simulink model "boost_and_two_level__1_sm_ehs"  (Simulink 8.4)
settings: Solver=ode3  SolverMode=SingleTasking  StartTime=0.0  StopTime=inf  FixedStep=2e-05  RelTol=1e-3
PostLoadFcn:
  | Ts = 20e-6;
InitFcn:
  | Ts = 20e-6;
undefined symbols (not defined in the file or in its folder): another_event_name, my_event_name, SW01
libraries: powerlib_meascontrol x12, opal_lib x7, rteventslib x6, rtlab x4, simulink x3, cpuhilios_lib x3, rtio_opalrt_common x2, artemis x1, simulink_extras x1, cpuconverter_lib x1
settings Model: ARTEMISmethode_block_infos=$$__separator__$$boost_and_two_level__1_sm_ehs/ARTEMIS Guide$$__separator__$$  Creator=PYRobert  LastModifiedBy=jiang  BufferReuse=off
settings DataIOCC: SaveOutput=off  SignalLogging=off  SaveTime=off  SignalLoggingName=sigsOut
settings OptimizationCC: BlockReduction=off  OptimizeBlockIOStorage=off  BufferReuse=off  GlobalBufferReuse=off  ExpressionFolding=off  LocalBlockOutputs=off  InitFltsAndDblsToZero=on
settings DebuggingCC: SaveWithParameterizedLinksMsg=none  SignalResolutionControl=TryResolveAllWithWarning  SolverPrmCheckMsg=none  MultiTaskDSMMsg=warning  MultiTaskCondExecSysMsg=none
settings HardwareCC: TargetEndianess=LittleEndian  TargetHWDeviceType=MATLAB Host  ProdEqTarget=off
settings RTWCC: GenCodeOnly=on  IncludeERTFirstTime=on
settings GRTTargetCC: TargetFcnLib=ansi_tfl_tmw.mat
settings ConfigurationSet: Description=SimMechanics 2G

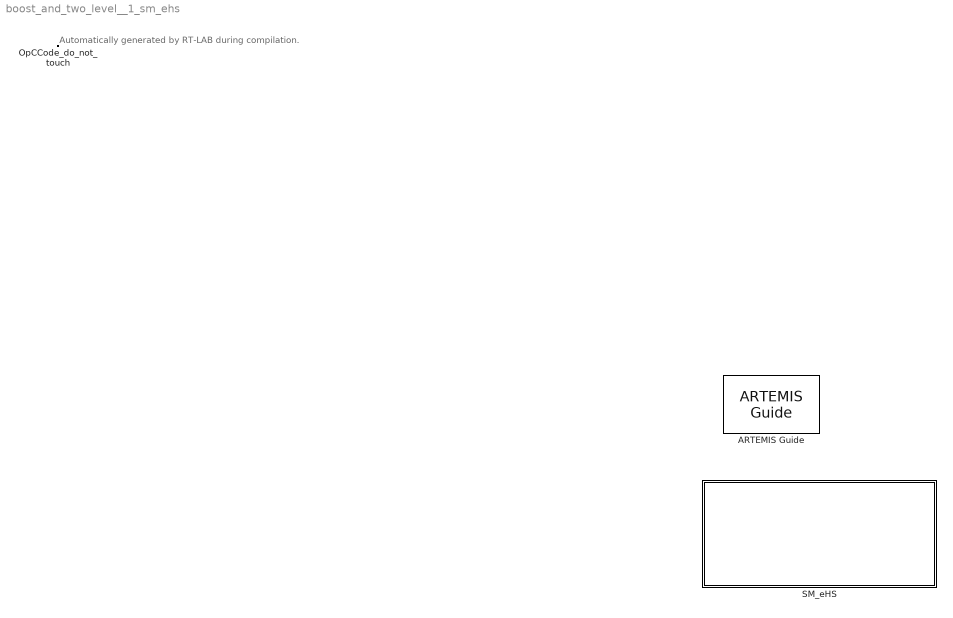
== system boost_and_two_level__1_sm_ehs ==
  note: Automatically generated by RT-LAB during compilation.
  ARTEMIS Guide : artemis/ARTEMIS/ARTEMIS Guide  Tag=FTSSmethode_opal_4hx0r99  Description=5.0_z1  lock=on  Ts=Ts  opt=art5  dyna=off  nb_perm=4  RT_fullcomp=off  ssn=on  ssn_itvc=off  ssn_ivic=off  ssn_ext=off  ssn_solver=Art5 with Backward Euler nodal interface  ssn_impulse=off  ssn_quasimpulse=off  ssn_impulse_loop=5  paraExtinctionThy=off  Thy_Impulse=on  dtc=Off  dtc_opt=normal  ao=on  simtype=off  ct_mac=off  lin_mov=off  lsp=[0.001 2]  spike_skip=Disabled  dtc_extra=1  dtc_sws=normal  dtc_pied=0.5  SPSRulesBlock=SPSRules  tre=on  ctmm=off  LF=off  dpl_type=ARTEMiS DPL  rlc_type=off  custom_type=off  para=on  ssn_ImpulseLoopBlockedStateUpdate=5  ssn_mov_iter_number=5  ssn_switch_iter_number=5
  OpCCode_do_not_touch : opal_lib/Communication/OpCCode  SystemSampleTime=-1
  SM_eHS : Subsystem

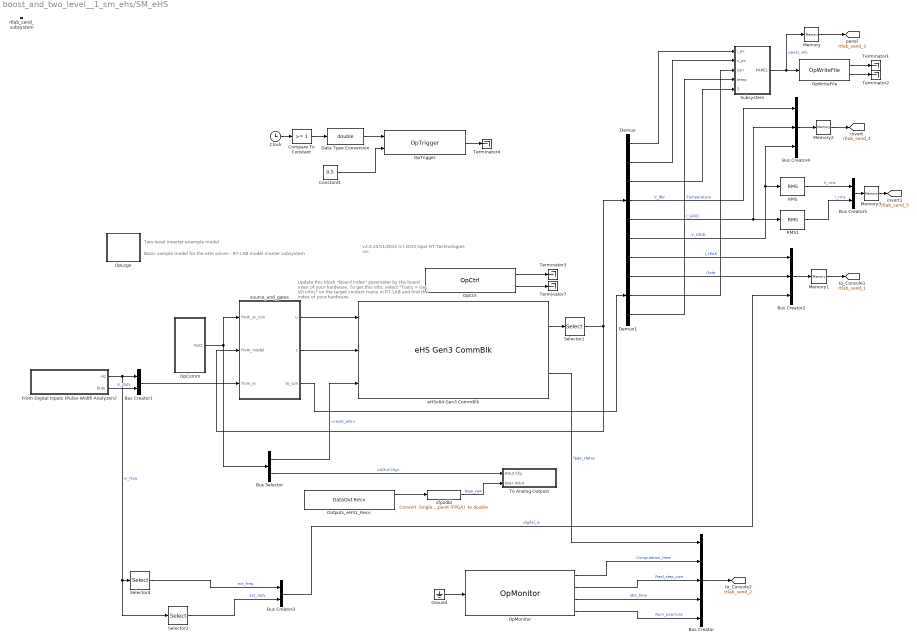
== system boost_and_two_level__1_sm_ehs/SM_eHS ==
  note: v2.0 25/11/2015
      | (c) 2015 Opal-RT Technologies inc.
  note: Two-level inverter example model
  note: Basic sample model for the eHS solver - RT-LAB model master subsystem
  note: Update this block "Board Index" parameter by the
      | board intex of your hardware. To get this info, select
      | "Tools > Get I/O infos" on the target context menu
      | in RT-LAB and find the index of your hardware.
  Bus Creator : BusCreator  Inputs=5
  Bus Creator1 : BusCreator  Inputs=2
  Bus Creator2 : BusCreator  Inputs=3
  Bus Creator3 : BusCreator  Inputs=2
  Bus Creator4 : BusCreator  Inputs=3
  Bus Creator5 : BusCreator  Inputs=2
  Bus Selector : BusSelector  OutputSignals=reset_ehs,AOut Cfg
  Clock : Clock
  Compare To Constant : simulink/Logic and Bit Operations/Compare To Constant  relop=>=  const=1  OutDataTypeStr=boolean
  Constant1 : Constant  Value=0.5
  Data Type Conversion : DataTypeConversion  OutDataTypeStr=double
  Demux : Demux  Outputs=7
  Demux1 : Demux  Outputs=3
  From Digital Inputs (Pulse-Width Analyzers) : Subsystem
  Ground : Ground
  Memory{,1..3} (4 alike) : Memory
  OpComm : Subsystem
      mask init:
      | opmaskdisplay('maskdisplay_block',gcb,'disp(''OpComm'')');
      mask Display:
      | patch([0 0.5 0.7 0],[1 1 0 0],[0.7 0.75 0.9]);
      | patch([1 0.53 0.73 1],[1 1 0 0],[1 0.8 0.7]);
      | plot([0 0 1 1 0],[0 1 1 0 0]);
      | disp('OpComm')
  OpCtrl : rtio_opalrt_common/OpCtrl  CtrlName='OpCtrl'  boardid=0  BitstreamFilename=MMPK7_1-EX-0001-2_3_2_19-300Series_eHSgen3_with_IOs-303-03.bin  numconfig=-1  mode=Master  externalClock=off  decimRtsi=0  calibIO=off  SampleTime=0  loadinport=-1  BoardType=MMPK7  SecondaryPresent=off  sync_type=Audio
  OpLogo : Subsystem
      mask Display:
      | opLogo = imread('efsOpLogo.tif','tif');
      | image(opLogo(:,:,1:3));
  OpMonitor : rtlab/Monitoring/OpMonitor  compute_time=on  real_step=on  idle_time=on  nb_overruns=on  user_time=off  user_name=my_event_name,another_event_name
  OpTrigger : rtlab/DataLogging/OpTrigger  Trig_Type=RISING OR FALLING EDGE  Trig_Offset=0  Acq_Group=26
  OpWriteFile : rtlab/DataLogging/OpWriteFile  Static_File=on  varname=opvar  Filename=myPV_inverter.mat  rtpath='./'  nrtpath='.\'  Acq_Group=26  file_size=1024*1024*1024  write_offline=off  Sim_Mode=off  Nb_Samples=4e5  Buffer_size=1024*1024
      settings: Decimation=100
  Outputs_eHS1_Recv : rtio_opalrt_common/DataOut Recv  CtrlName='OpCtrl'  FcnNos=2  width=7  portType=uint32  sampleTime=0  checkVersion=off  expectedId=0  expectedVersion=0  opComp=>=
      settings: AttributesFormatString=%<CtrlName>
  RMS : powerlib_meascontrol/Measurements/RMS  TrueRMS=on  Freq=50  RMSInit=0  Ts=0
  RMS1 : powerlib_meascontrol/Measurements/RMS  TrueRMS=on  Freq=50  RMSInit=0  Ts=0
  Selector1 : Selector  Indices=[1:7]
  Selector2 : Selector  InputPortWidth=2  Indices=[2]
  Selector4 : Selector  InputPortWidth=2  Indices=[1]
  Subsystem : Subsystem
  Terminator{1..4,7} (5 alike) : Terminator
  To Analog Outputs : Subsystem
  eHSx64 Gen3 CommBlk : cpuconverter_lib/eHS Gen3 CommBlk  GenMat=off  solver_size=x64  circuit_mtx1=my_pv_sys_fpga.mdl  Ts_eHS_1_explicit=on  Ts_eHS_1=2.5e-07  SimeHS1=off  ShowAdv1=on  gs1=0.076389  v_init1=400*ones(1,24)  i_init1=zeros(1,24)  netlist_name=my_pv_sys_fpga.mdl  ts_min=2.05e-07  nb_u=3  input_names=|  nb_sw=4  switches_names=SW01-04_01 | SW01-04_02 | SW01-04_03 | SW01-04_04  nb_y=7  output_names=Y01 IPANEL I | Y02 VPANEL U | Y03 VPH U | Y04 VINV U | Y05 IGRID I | Y06 VGRID U | Y07 IG I  nb_nsd=12  Input_config1_popup=Constant from RT-LAB block (all)  input_config_1="[zeros(32,1)  (0:31)']"  input_nb_auto=on  input_nb=3  UseSWG=off  SWGPortNbs=3  Pulse_ctrl1_popup=Independent setting for each element  GateCtrlSelPanel=off  Pulse_ctrl1=[zeros(72,1) (0:71)']  Polarity1_popup=Active-high (all)  Polarity1=zeros(1,72)  pulse_nb=8  rte_pulse_nb=SW01-08  nb_event=4  static_pulse=none  scn_en=off  xls_file=diode_bridge.xls  scn_cmd=do nothing  xls_page=1  nscn_max=102  nscn_used=1  scn_log_en=on  CtrlName='OpCtrl'  Ts=Ts  PortNbs=[1 2 1 2:1:2+8 1]  blkid1=0
      | U01
      | 14,400 V | U02 IPH
      |  | U03 ID
      settings: AttributesFormatString=%<CtrlName>
  rtlab_send_subsystem : Subsystem  Priority=-100
      mask Display: text(0,0,'');
  sfp2dbl : rtlab/Miscellaneous/Convert  Single floating-point (FPGA)  to double
  source_and_gates : Subsystem
  tag scope: rtlab_send_1=global, rtlab_send_2=global, rtlab_send_3=global, rtlab_send_4=global, rtlab_send_5=global
  wires:
  OpComm/1(Out1) -> Bus Selector/1, source_and_gates/1(from_sc_con)
  OpCtrl/1 -> Terminator3/1
  OpCtrl/2 -> Terminator7/1
  source_and_gates/1(u) -> eHSx64 Gen3 CommBlk/1
  source_and_gates/2(c) -> eHSx64 Gen3 CommBlk/2
  eHSx64 Gen3 CommBlk/1 -> Selector1/1
  Outputs_eHS1_Recv/1 -> sfp2dbl/1
  Bus Selector/1 -> eHSx64 Gen3 CommBlk/3  "<reset_ehs>"
  Selector1/1 -> Demux/1, source_and_gates/2(from_model)
  OpWriteFile/1 -> Terminator1/1
  OpWriteFile/2 -> Terminator2/1
  Clock/1 -> Compare To Constant/1
  Constant1/1 -> OpTrigger/2
  OpTrigger/1 -> Terminator4/1
  Compare To Constant/1 -> Data Type Conversion/1
  Data Type Conversion/1 -> OpTrigger/1
  Ground/1 -> OpMonitor/1
  Bus Creator/1 -> [rtlab_send_2]
  sfp2dbl/1 -> To Analog Outputs/2(User AOut)  "fpga_raw"
  OpMonitor/4 -> Bus Creator/5  "Num_overruns"
  OpMonitor/3 -> Bus Creator/4  "Idle_time"
  OpMonitor/2 -> Bus Creator/3  "Real_step_size"
  OpMonitor/1 -> Bus Creator/2  "Computation_time"
  Subsystem/1(PANEL) -> Memory/1, OpWriteFile/1  "panel_info"
  Bus Selector/2 -> To Analog Outputs/1(AOut Cfg)  "<AOut Cfg>"
  Demux/1 -> Subsystem/1(i_pv)
  Demux/2 -> Subsystem/2(v_pv)
  Demux/4 -> Bus Creator4/1  "V_INV"
  Demux/3 -> Subsystem/5(i_diode)
  Demux/5 -> RMS1/1, Bus Creator4/2  "I_GRID"
  Demux/6 -> RMS/1, Bus Creator4/3  "V_GRID"
  Demux/7 -> Bus Creator2/1  "I_LEAK"
  source_and_gates/3(to_con) -> Demux1/1
  Demux1/3 -> Subsystem/4(temp)  "Temperature"
  Demux1/1 -> Bus Creator2/2  "Gate"
  Demux1/2 -> Subsystem/3(sun)
  Bus Creator2/1 -> Memory1/1
  From Digital Inputs (Pulse-Width Analyzers)/1(Hz) -> Selector2/1, Selector4/1, Bus Creator1/1  "in_freq"
  From Digital Inputs (Pulse-Width Analyzers)/2(Duty) -> Bus Creator1/2  "in_duty"
  Bus Creator1/1 -> source_and_gates/3(from_io)
  Selector4/1 -> Bus Creator3/1  "ext_freq"
  Bus Creator3/1 -> Bus Creator2/3  "digital_in"
  eHSx64 Gen3 CommBlk/2 -> Bus Creator/1  "fpga_status"
  Memory/1 -> [rtlab_send_3]
  Memory1/1 -> [rtlab_send_1]
  Memory2/1 -> [rtlab_send_4]
  Bus Creator4/1 -> Memory2/1
  RMS/1 -> Bus Creator5/1  "V_rms"
  RMS1/1 -> Bus Creator5/2  "I_rms"
  Bus Creator5/1 -> Memory3/1
  Memory3/1 -> [rtlab_send_5]
  Selector2/1 -> Bus Creator3/2  "ext_duty"

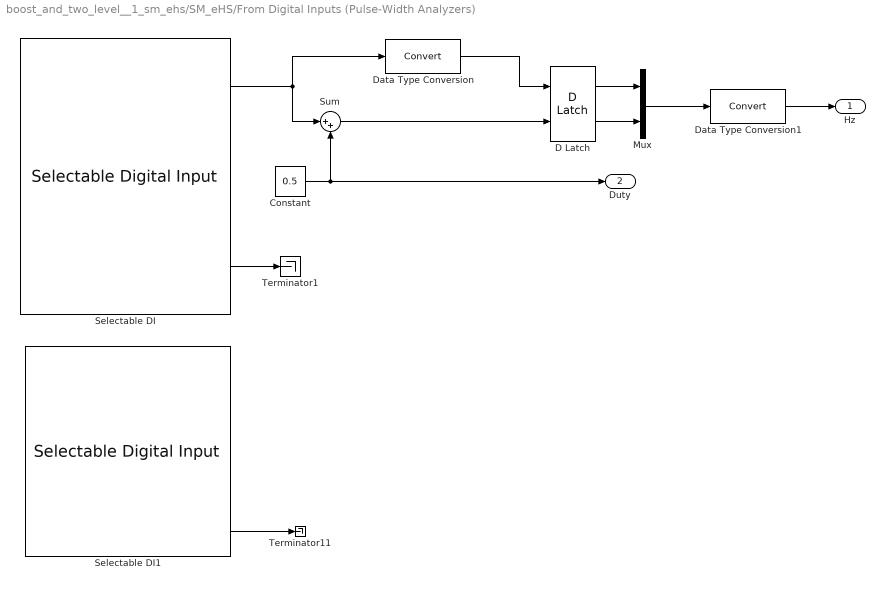
== system boost_and_two_level__1_sm_ehs/SM_eHS/From Digital Inputs (Pulse-Width Analyzers) ==
  Constant : Constant  Value=0.5
  D Latch : simulink_extras/Flip Flops/D Latch
  Data Type Conversion : DataTypeConversion
  Data Type Conversion1 : DataTypeConversion
  Mux : Mux  Inputs=2
  Selectable DI : cpuhilios_lib/Selectable Digital Input  CtrlName='OpCtrl'  DataInPortNumber=5  LoadInPortNumber=13  IOTypeSel=Event Detector  FcnNos=Slot 1 Module A Subsection 1  maxcount=8  count=1  width=1  timeUnit=Time ratio  sampleTime=0
      settings: AttributesFormatString=%<CtrlName>
  Selectable DI1 : cpuhilios_lib/Selectable Digital Input  CtrlName='OpCtrl'  DataInPortNumber=6  LoadInPortNumber=14  IOTypeSel=Event Detector  FcnNos=Slot 1 Module A Subsection 2  maxcount=8  count=8  width=0  timeUnit=Time ratio  sampleTime=0
      settings: AttributesFormatString=%<CtrlName>
  Sum : Sum  Inputs=|++
  Terminator1 : Terminator
  Terminator11 : Terminator
  Hz : Outport
  Duty : Outport  Port=2
  wires:
  Selectable DI1/17 -> Terminator11/1
  Selectable DI/3 -> Terminator1/1
  D Latch/1 -> Mux/1
  D Latch/2 -> Mux/2
  Mux/1 -> Data Type Conversion1/1
  Selectable DI/1 -> Sum/1, Data Type Conversion/1
  Constant/1 -> Duty/1, Sum/2
  Data Type Conversion/1 -> D Latch/1
  Sum/1 -> D Latch/2
  Data Type Conversion1/1 -> Hz/1

== system boost_and_two_level__1_sm_ehs/SM_eHS/OpComm ==
  Demux : Demux  Outputs=[165]
  Receive : opal_lib/Communication/OpRecPar FromNT  Data_width=165  InitialConditions=[1000;25;1;0;49;48;52;53;53;9;1;3;12;13;0;2;48;49;50;51;48;49;50;51;52;53;54;54;56;57;58;59;60;61;62;63;0.0066;0.33;0.066;0.004125;0.0048529;1;0.005;0.005;0.1;0.1;0.1;0.1;0.005;0.1;0.1;0.1;1;1;1;1;1;1;1;1;1;1;1;1;1;1;1;1;0;0;1.65;1.65;1.65;0;0;0;0;0;0;0;0;0;0;0;0;0;0;0;0;0;0;0;0;0;0;0;0;0;0;0;3.3;3.3;3.3;3.3;3.3;5;5;5;5;5;5;5;16;16;16;16;16;16;16;16;16;16;16;16;16;16;16;16;16;16;16;16;0;0;0;0;0;-5;-5;-5;-5;-5;-5;-5;-16;-16;-16;-16;-16;-16;-16;-16;-16;-16;-16;-16;-16;-16;-16;-16;-16;-16;-16;-16;2]
  busStruct : Subsystem
  Out1 : Outport
  wires:
  Demux/1 -> busStruct/1(In1)
  busStruct/1(Out1) -> Out1/1
  Receive/1 -> Demux/1

== system boost_and_two_level__1_sm_ehs/SM_eHS/OpLogo ==

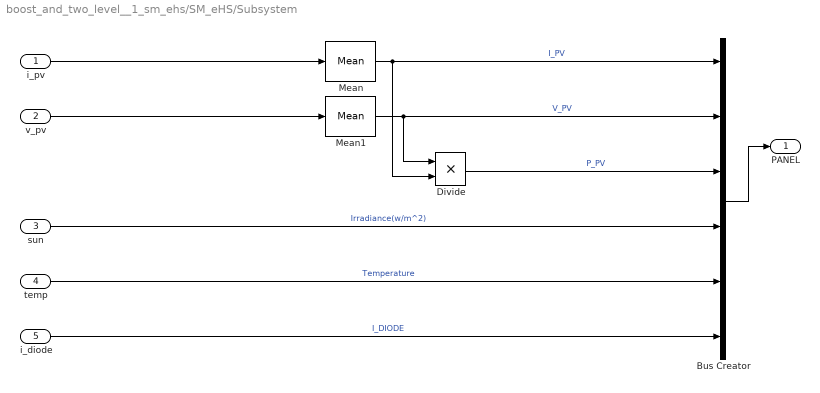
== system boost_and_two_level__1_sm_ehs/SM_eHS/Subsystem ==
  i_pv : Inport
  v_pv : Inport  Port=2
  sun : Inport  Port=3
  temp : Inport  Port=4
  i_diode : Inport  Port=5
  Bus Creator : BusCreator  Inputs=6
  Divide : Product  Inputs=**
  Mean : powerlib_meascontrol/Measurements/Mean  Freq=50  Vinit=0  Ts=0
  Mean1 : powerlib_meascontrol/Measurements/Mean  Freq=50  Vinit=0  Ts=0
  PANEL : Outport
  wires:
  Divide/1 -> Bus Creator/3  "P_PV"
  Mean/1 -> Divide/2, Bus Creator/1  "I_PV"
  Mean1/1 -> Divide/1, Bus Creator/2  "V_PV"
  sun/1 -> Bus Creator/4  "Irradiance(w/m^2)"
  i_pv/1 -> Mean/1
  v_pv/1 -> Mean1/1
  Bus Creator/1 -> PANEL/1
  temp/1 -> Bus Creator/5  "Temperature"
  i_diode/1 -> Bus Creator/6  "I_DIODE"

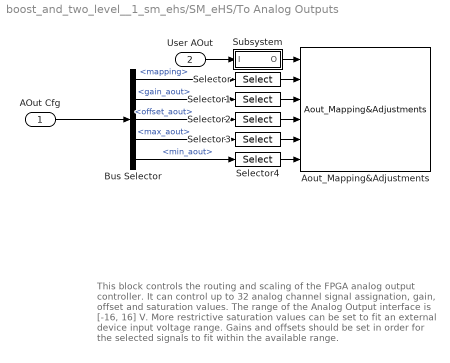
== system boost_and_two_level__1_sm_ehs/SM_eHS/To Analog Outputs ==
  note: This block controls the routing and scaling of the FPGA analog
      | output controller.
      |
      |  It can control up to 32 analog channel signal assignation, gain,
      | offset and saturation values.
      |
      | The range of the Analog Output interface is [-16, 16] V.  More
      | restrictive saturation values can be set to fit an external device
      | input voltage range. Gains and offsets should be set in order for
      | the selected signals to fit within the available range.
  AOut Cfg : Inport
  User AOut : Inport  Port=2
  Aout_Mapping&Adjustments : cpuhilios_lib/Aout_Mapping&Adjustments  ChNum=16 (1 Aout mezz)  UserAoutNum=16  block_index=0  DataInId=15  LoadInId=4  CtrlerName='OpCtrl'
      settings: AttributesFormatString=%<CtrlerName>
  Bus Selector : BusSelector  OutputSignals=mapping,gain_aout,offset_aout,max_aout,min_aout
  Selector{,1..4} (5 alike) : Selector  InputPortWidth=32  Indices=[1:1:16]
  Subsystem : Subsystem
  wires:
  User AOut/1 -> Subsystem/1(I)
  Bus Selector/2 -> Selector1/1  "<gain_aout>"
  Bus Selector/5 -> Selector4/1  "<min_aout>"
  Bus Selector/4 -> Selector3/1  "<max_aout>"
  Bus Selector/1 -> Selector/1  "<mapping>"
  Bus Selector/3 -> Selector2/1  "<offset_aout>"
  AOut Cfg/1 -> Bus Selector/1
  Subsystem/1(O) -> Aout_Mapping&Adjustments/1
  Selector/1 -> Aout_Mapping&Adjustments/2
  Selector1/1 -> Aout_Mapping&Adjustments/3
  Selector2/1 -> Aout_Mapping&Adjustments/4
  Selector3/1 -> Aout_Mapping&Adjustments/5
  Selector4/1 -> Aout_Mapping&Adjustments/6

== system boost_and_two_level__1_sm_ehs/SM_eHS/rtlab_send_subsystem ==
  Subsystem1 : Subsystem
  Subsystem2 : Subsystem
  Subsystem3 : Subsystem
  Subsystem4 : Subsystem
  Subsystem5 : Subsystem
  wires:
  [rtlab_send_1] -> Subsystem1/1(In1)
  [rtlab_send_2] -> Subsystem2/1(In1)
  [rtlab_send_4] -> Subsystem3/1(In1)
  [rtlab_send_3] -> Subsystem4/1(In1)
  [rtlab_send_5] -> Subsystem5/1(In1)

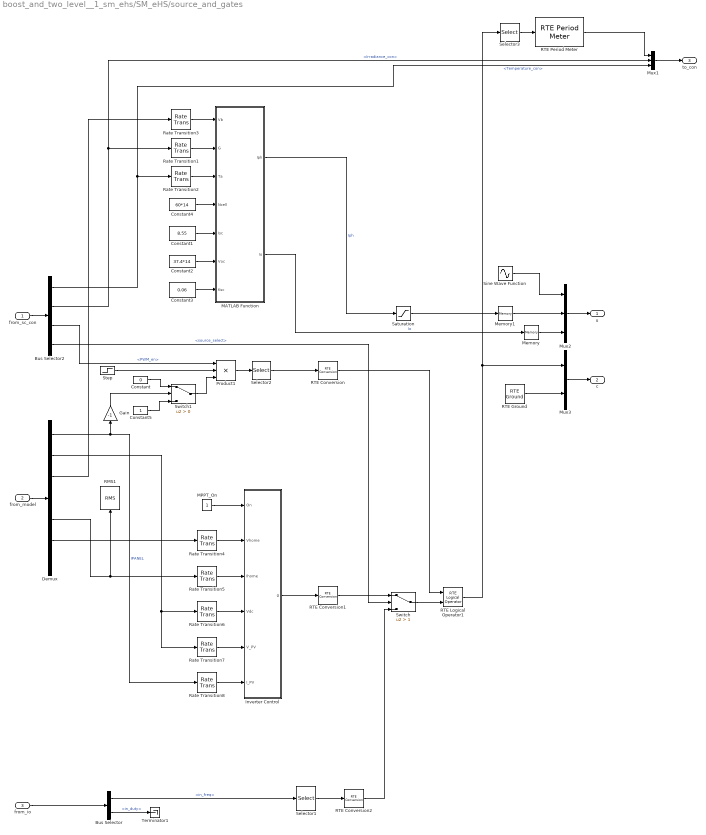
== system boost_and_two_level__1_sm_ehs/SM_eHS/source_and_gates ==
  from_sc_con : Inport
  from_model : Inport  Port=2
  from_io : Inport  Port=3
  Bus Selector : BusSelector  OutputSignals=in_freq,in_duty
  Bus Selector2 : BusSelector  OutputSignals=Temperature_con,Irradiance_con,PWM_en,source_select
  Constant : Constant  Value=0
  Constant1 : Constant  Value=8.55
  Constant2 : Constant  Value=37.4*14
  Constant3 : Constant  Value=0.06
  Constant4 : Constant  Value=60*14
  Constant5 : Constant
  Demux : Demux  Outputs=7
  Gain : Gain  Gain=-1
  Inverter Control : Subsystem  mask(Inverter Control){Pnom=3500, Fnom=50, Vnom_prim=240, Vnom_dc=400, Increment_MPPT=0.003, Limits_MPPT=[ 450 375 ], Vdc_ref_Init=425, Kp_VDCreg=12, Ki_VDCreg=200, Kp_Ireg=0.15, Ki_Ireg=6.6, RLff=[ 0.002 0.20 ], Fc=8000, PWMmode12=Bipolar, Ts_Control=Ts, Ts_PWMgenerator=Ts}
      mask prompts: Pnom "Power (VA)"; Fnom "Frequency (Hz)"; Vnom_prim "Primary voltage (Vrms LL)"; Vnom_dc "DC voltage (V)"; Increment_MPPT "Output increment (V)"; Limits_MPPT "Output limits [ Upper  Lower ]"; Vdc_ref_Init "Output initial value (V)"; Kp_VDCreg "Proportional gain"; Ki_VDCreg "Integral gain"; Kp_Ireg "Proportional gain"; Ki_Ireg "Integral gain"; RLff "Feedforward Values [Rff Lff] (pu)"; Fc "Carrier frequency (Hz)"; PWMmode12 "PWM method"; Ts_Control "Control systems"; Ts_PWMgenerator "PWM generator"
      mask help:
      | The main components of the Inverter Control are:
      | 1. PLL & Measurements
      | 2. Maximum Power Point Tracker System (MPPT) using a Perturb & Observe algorithm
      | 3. DC Voltage Regulator
      | 4. Current Regulator
      | 5. PWM Modulator
      mask TypeOptions PWMmode12: Unipolar | Bipolar
      mask Display:
      | blockName=gcb;
      | if PWMmode12==1
      |     set_param([blockName,'/','PWM_Generator'],'ModulatorType','Single-phase full-bridge (4 pulses)')
      | else
      |     set_param([blockName,'/','PWM_Generator'],'ModulatorType','Single-phase full-bridge - Bipolar modulation (4 pulses)')
      | end
  MATLAB Function : MATLAB Function  TreatAsAtomicUnit=on
  MPPT_On : Constant
  Memory : Memory  InheritSampleTime=on  LinearizeAsDelay=on
  Memory1 : Memory  InheritSampleTime=on  LinearizeAsDelay=on
  Mux1 : Mux  Inputs=3
  Mux2 : Mux  Inputs=3
  Mux3 : Mux  Inputs=2
  Product1 : Product  Inputs=3  RndMeth=Zero
  RMS1 : powerlib_meascontrol/Measurements/RMS  TrueRMS=on  Freq=50  RMSInit=0  Ts=0
  RTE Conversion : rteventslib/Signal Attributes/RTE Conversion  inputdatatype=Double  outputdatatype=RTE Boolean  compensation=Enabled  nbMaxEvents=100  sampleTime=Ts
  RTE Conversion1 : rteventslib/Signal Attributes/RTE Conversion  inputdatatype=Double  outputdatatype=RTE Boolean  compensation=Enabled  nbMaxEvents=4  sampleTime=Ts
  RTE Conversion2 : rteventslib/Signal Attributes/RTE Conversion  inputdatatype=Double  outputdatatype=RTE Boolean  compensation=Enabled  nbMaxEvents=4  sampleTime=Ts
  RTE Ground : rteventslib/Sources/RTE Ground  SampleTime=Ts
  RTE Logical Operator1 : rteventslib/Math Operations/RTE Logical Operator  LogicalOperator=AND  NbrInput=2  NbrMaxEvents=255
  RTE Period Meter : rteventslib/Signal Attributes/RTE Period Meter  Period=off  Frequency=off  EdgeType=Rising edges  TOn=off  TOff=off  DutyCycle=on  DuringType=Signal period  MinimumFrequency=0
  Rate Transition1 : RateTransition  X0=1000
  Rate Transition2 : RateTransition  X0=25
  Rate Transition3 : RateTransition  X0=400
  Rate Transition4 : RateTransition
  Rate Transition5 : RateTransition
  Rate Transition6 : RateTransition  X0=400
  Rate Transition7 : RateTransition  X0=400
  Rate Transition8 : RateTransition
  Saturation : Saturate  UpperLimit=10  LowerLimit=0
  Selector1 : Selector  InputPortWidth=2  Indices=[1 2 2 1]
  Selector2 : Selector  InputPortWidth=1  Indices=[ones(1,4)*1]
  Selector3 : Selector  Indices=[1]
  Sine Wave Function : Sin  Amplitude=14400*sqrt(2)  Frequency=50*2*pi  SampleTime=0
  Step : Step  Time=0.05  SampleTime=Ts
  Switch : Switch  Criteria=u2 > Threshold  Threshold=1
  Switch1 : Switch  Criteria=u2 > Threshold
  Terminator1 : Terminator
  u : Outport
  c : Outport  Port=2
  to_con : Outport  Port=3
  wires:
  Bus Selector2/3 -> Product1/1  "<PWM_en>"
  Step/1 -> Product1/2
  Product1/1 -> Selector2/1
  Mux2/1 -> u/1
  from_sc_con/1 -> Bus Selector2/1
  MPPT_On/1 -> Inverter Control/1(On)
  Constant4/1 -> MATLAB Function/4(Ncell)
  Constant1/1 -> MATLAB Function/5(Isc)
  Constant2/1 -> MATLAB Function/6(Voc)
  Constant3/1 -> MATLAB Function/7(Ksc)
  from_model/1 -> Demux/1
  Demux/1 -> Gain/1, Rate Transition8/1  "IPANEL"
  Demux/2 -> Rate Transition7/1, Rate Transition6/1
  Demux/6 -> Rate Transition4/1
  Demux/5 -> RMS1/1, Rate Transition5/1
  Mux1/1 -> to_con/1
  RTE Ground/1 -> Mux3/2
  Mux3/1 -> c/1
  Sine Wave Function/1 -> Mux2/1
  MATLAB Function/2(Io) -> Memory/1  "Io"
  Saturation/1 -> Memory1/1
  MATLAB Function/1(Iph) -> Saturation/1  "Iph"
  Memory1/1 -> Mux2/2
  Memory/1 -> Mux2/3
  Rate Transition3/1 -> MATLAB Function/1(Vb)
  Rate Transition1/1 -> MATLAB Function/2(G)
  Rate Transition2/1 -> MATLAB Function/3(Ta)
  Bus Selector2/2 -> Mux1/2, Rate Transition1/1  "<Irradiance_con>"
  Bus Selector2/1 -> Rate Transition2/1, Mux1/3  "<Temperature_con>"
  Demux/3 -> Rate Transition3/1
  Rate Transition4/1 -> Inverter Control/2(Vhome)
  Rate Transition5/1 -> Inverter Control/3(Ihome)
  Rate Transition6/1 -> Inverter Control/4(Vdc)
  Rate Transition7/1 -> Inverter Control/5(V_PV)
  Rate Transition8/1 -> Inverter Control/6(I_PV)
  Inverter Control/1(g) -> RTE Conversion1/1
  Selector3/1 -> RTE Period Meter/1
  Bus Selector/1 -> Selector1/1  "<in_freq>"
  from_io/1 -> Bus Selector/1
  Bus Selector/2 -> Terminator1/1  "<in_duty>"
  Bus Selector2/4 -> Switch/2  "<source_select>"
  RTE Conversion2/1 -> Switch/3
  RTE Period Meter/1 -> Mux1/1
  RTE Conversion1/1 -> Switch/1
  Selector2/1 -> RTE Conversion/1
  RTE Conversion/1 -> RTE Logical Operator1/1
  Switch/1 -> RTE Logical Operator1/2
  RTE Logical Operator1/1 -> Selector3/1, Mux3/1
  Selector1/1 -> RTE Conversion2/1
  Switch1/1 -> Product1/3
  Constant/1 -> Switch1/1
  Constant5/1 -> Switch1/3
  Gain/1 -> Switch1/2

== system boost_and_two_level__1_sm_ehs/SM_eHS/OpComm/busStruct ==
  In1 : Inport
  Sub1 : Subsystem
  Out1 : Outport
  wires:
  Sub1/1(goto_global) -> Out1/1
  In1/1 -> Sub1/1(from_global)

== system boost_and_two_level__1_sm_ehs/SM_eHS/To Analog Outputs/Subsystem ==
  I : Inport
  Constant : Constant  Value=ones(1,9)
  Mux : Mux  Inputs=2
  O : Outport
  wires:
  Constant/1 -> Mux/2
  I/1 -> Mux/1
  Mux/1 -> O/1

== system boost_and_two_level__1_sm_ehs/SM_eHS/rtlab_send_subsystem/Subsystem1 ==
  In1 : Inport
  Mux : Mux  Inputs=1
  Send1 : opal_lib/Communication/OpSendToNT  Acqu_group=1
  wires:
  Mux/1 -> Send1/1
  In1/1 -> Mux/1

== system boost_and_two_level__1_sm_ehs/SM_eHS/rtlab_send_subsystem/Subsystem2 ==
  In1 : Inport
  Mux : Mux  Inputs=1
  Send2 : opal_lib/Communication/OpSendToNT  Acqu_group=2
  wires:
  Mux/1 -> Send2/1
  In1/1 -> Mux/1

== system boost_and_two_level__1_sm_ehs/SM_eHS/rtlab_send_subsystem/Subsystem3 ==
  In1 : Inport
  Mux : Mux  Inputs=1
  Send3 : opal_lib/Communication/OpSendToNT  Acqu_group=4
  wires:
  Mux/1 -> Send3/1
  In1/1 -> Mux/1

== system boost_and_two_level__1_sm_ehs/SM_eHS/rtlab_send_subsystem/Subsystem4 ==
  In1 : Inport
  Mux : Mux  Inputs=1
  Send4 : opal_lib/Communication/OpSendToNT  Acqu_group=3
  wires:
  Mux/1 -> Send4/1
  In1/1 -> Mux/1

== system boost_and_two_level__1_sm_ehs/SM_eHS/rtlab_send_subsystem/Subsystem5 ==
  In1 : Inport
  Mux : Mux  Inputs=1
  Send5 : opal_lib/Communication/OpSendToNT  Acqu_group=5
  wires:
  Mux/1 -> Send5/1
  In1/1 -> Mux/1

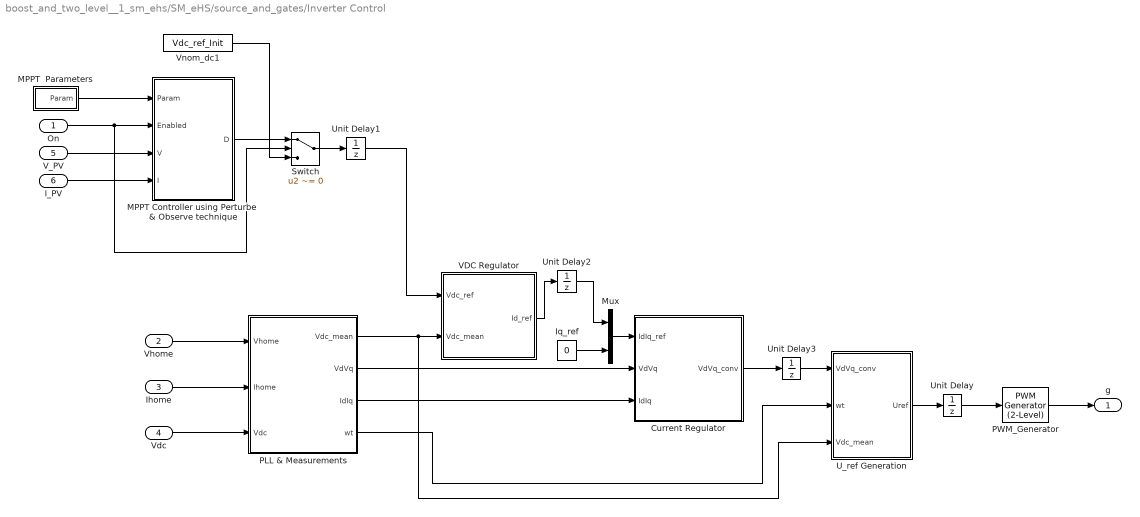
== system boost_and_two_level__1_sm_ehs/SM_eHS/source_and_gates/Inverter Control ==
  On : Inport  PortDimensions=1
  Vhome : Inport  Port=2  PortDimensions=1
  Ihome : Inport  Port=3  PortDimensions=1
  Vdc : Inport  Port=4  PortDimensions=1
  V_PV : Inport  Port=5  PortDimensions=1
  I_PV : Inport  Port=6  PortDimensions=1
  Current Regulator : Subsystem
  Iq_ref : Constant  Value=0
  MPPT  Parameters : Subsystem
  "MPPT Controller using Perturbe  & Observe technique  " : MATLAB Function  TreatAsAtomicUnit=on
  Mux : Mux  Inputs=2
  PLL & Measurements : Subsystem
  PWM_Generator : powerlib_meascontrol/Pulse & Signal Generators/PWM Generator (2-Level)  ModulatorType=Single-phase full-bridge - Bipolar modulation (4 pulses)  ModulatorMode=Unsynchronized  Fc=Fc  Pc=90  nF=27  MinMax="[ -1  1 ]"  SamplingTechnique=Natural  ModulatingSignals=off  m=0.8  Freq=60  Phase=0  Ts=Ts_PWMgenerator  ShowCarrierOutport=off
      settings: AttributesFormatString=%<ModulatorType>
  Switch : Switch  Criteria=u2 ~= 0
  "U_ref Generation " : Subsystem
  Unit Delay : UnitDelay  InitialCondition=0.1684  SampleTime=Ts_Control
  Unit Delay1 : UnitDelay  SampleTime=Ts_Control
  Unit Delay2 : UnitDelay  SampleTime=Ts_Control
  Unit Delay3 : UnitDelay  SampleTime=Ts_Control
  VDC Regulator : Subsystem
  Vnom_dc1 : Constant  Value=Vdc_ref_Init
  g : Outport
  wires:
  Iq_ref/1 -> Mux/2
  Vhome/1 -> PLL & Measurements/1(Vhome)
  Ihome/1 -> PLL & Measurements/2(Ihome)
  V_PV/1 -> "MPPT Controller using Perturbe  & Observe technique  "/3(V)
  I_PV/1 -> "MPPT Controller using Perturbe  & Observe technique  "/4(I)
  MPPT  Parameters/1(Param) -> "MPPT Controller using Perturbe  & Observe technique  "/1(Param)
  On/1 -> "MPPT Controller using Perturbe  & Observe technique  "/2(Enabled), Switch/2
  "MPPT Controller using Perturbe  & Observe technique  "/1(D) -> Switch/1
  Vdc/1 -> PLL & Measurements/3(Vdc)
  Vnom_dc1/1 -> Switch/3
  PLL & Measurements/2(VdVq) -> Current Regulator/2(VdVq)
  PLL & Measurements/3(IdIq) -> Current Regulator/3(IdIq)
  Mux/1 -> Current Regulator/1(IdIq_ref)
  PLL & Measurements/1(Vdc_mean) -> "U_ref Generation "/3(Vdc_mean), VDC Regulator/2(Vdc_mean)
  PLL & Measurements/4(wt) -> "U_ref Generation "/2(wt)
  "U_ref Generation "/1(Uref) -> Unit Delay/1
  Switch/1 -> Unit Delay1/1
  Unit Delay1/1 -> VDC Regulator/1(Vdc_ref)
  VDC Regulator/1(Id_ref) -> Unit Delay2/1
  Unit Delay2/1 -> Mux/1
  Current Regulator/1(VdVq_conv) -> Unit Delay3/1
  Unit Delay3/1 -> "U_ref Generation "/1(VdVq_conv)
  PWM_Generator/1 -> g/1
  Unit Delay/1 -> PWM_Generator/1

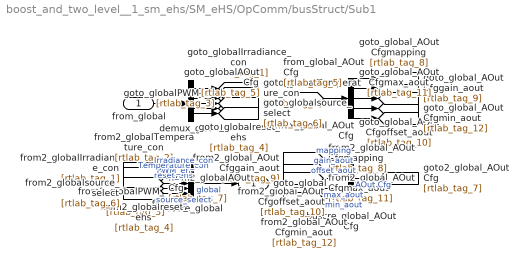
== system boost_and_two_level__1_sm_ehs/SM_eHS/OpComm/busStruct/Sub1 ==
  from_global : Inport
  buscre_global : BusCreator  Inputs=6
  buscre_global_AOut Cfg : BusCreator  Inputs=5
  demux_global : Demux  Outputs="[1    1    1    1  160    1]"
  demux_global_AOut Cfg : Demux  Outputs="[32  32  32  32  32]"
  goto_global : Outport
  wires:
  buscre_global_AOut Cfg/1 -> [rtlab_tag_7]  "AOut Cfg"
  [rtlab_tag_12] -> buscre_global_AOut Cfg/5  "min_aout"
  [rtlab_tag_11] -> buscre_global_AOut Cfg/4  "max_aout"
  [rtlab_tag_10] -> buscre_global_AOut Cfg/3  "offset_aout"
  [rtlab_tag_9] -> buscre_global_AOut Cfg/2  "gain_aout"
  [rtlab_tag_8] -> buscre_global_AOut Cfg/1  "mapping"
  demux_global_AOut Cfg/5 -> [rtlab_tag_12]
  demux_global_AOut Cfg/4 -> [rtlab_tag_11]
  demux_global_AOut Cfg/3 -> [rtlab_tag_10]
  demux_global_AOut Cfg/2 -> [rtlab_tag_9]
  demux_global_AOut Cfg/1 -> [rtlab_tag_8]
  [rtlab_tag_5] -> demux_global_AOut Cfg/1
  buscre_global/1 -> goto_global/1  "global"
  [rtlab_tag_6] -> buscre_global/6  "source_select"
  [rtlab_tag_7] -> buscre_global/5
  [rtlab_tag_4] -> buscre_global/4  "reset_ehs"
  [rtlab_tag_3] -> buscre_global/3  "PWM_en"
  [rtlab_tag_2] -> buscre_global/2  "Temperature_con"
  [rtlab_tag_1] -> buscre_global/1  "Irradiance_con"
  demux_global/6 -> [rtlab_tag_6]
  demux_global/5 -> [rtlab_tag_5]
  demux_global/4 -> [rtlab_tag_4]
  demux_global/3 -> [rtlab_tag_3]
  demux_global/2 -> [rtlab_tag_2]
  demux_global/1 -> [rtlab_tag_1]
  from_global/1 -> demux_global/1

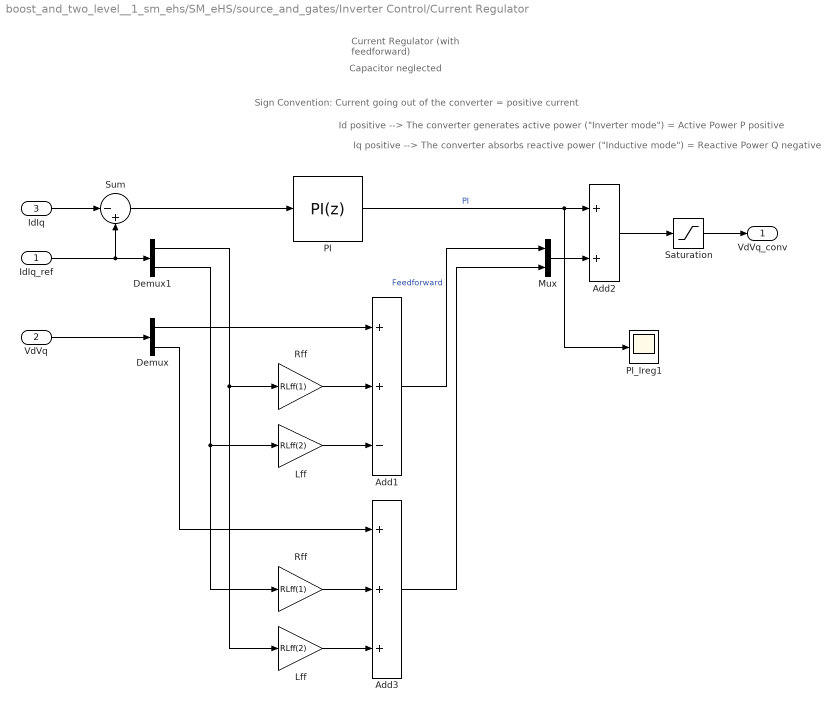
== system boost_and_two_level__1_sm_ehs/SM_eHS/source_and_gates/Inverter Control/Current Regulator ==
  note: Id positive --> The converter generates active power ("Inverter mode") = Active Power P positive
  note: Iq positive --> The converter absorbs reactive power ("Inductive mode") = Reactive Power Q negative
  note: Sign Convention: Current going out of the converter = positive current
  note: Current Regulator
      | (with feedforward)
  note: Capacitor neglected
  IdIq_ref : Inport  PortDimensions=2
  VdVq : Inport  Port=2  PortDimensions=2
  IdIq : Inport  Port=3  PortDimensions=2
  Add1 : Sum  Inputs=++-
  Add2 : Sum
  Add3 : Sum  Inputs=+++
  Demux : Demux  Outputs=2
  Demux1 : Demux  Outputs=2
  Lff : Gain  Gain=RLff(2)  SaturateOnIntegerOverflow=on  OutDataTypeStr=Inherit: Same as input  ParamDataTypeStr=Inherit: Same as input
  "Lff  " : Gain  Gain=RLff(2)  SaturateOnIntegerOverflow=on  OutDataTypeStr=Inherit: Same as input  ParamDataTypeStr=Inherit: Same as input
  Mux : Mux  Inputs=2
  PI : simulink/Continuous/PID Controller  Controller=PI  TimeDomain=Discrete-time  SampleTime=Ts_Control  IntegratorMethod=Forward Euler  FilterMethod=Forward Euler  Form=Parallel  P=Kp_Ireg  I=Ki_Ireg  D=0  N=100  InitialConditionSource=internal  InitialConditionForIntegrator=0  InitialConditionForFilter=0  ExternalReset=none  LimitOutput=on  UpperSaturationLimit=1.5  LowerSaturationLimit=-1.5  LinearizeAsGain=off  AntiWindupMode=none  Kb=1  TrackingMode=off  Kt=1  PParamMin=[]  PParamMax=[]  IParamMin=[]  IParamMax=[]  DParamMin=[]  DParamMax=[]  NParamMin=[]  NParamMax=[]  KbParamMin=[]  KbParamMax=[]  KtParamMin=[]  KtParamMax=[]  POutMin=[]  POutMax=[]  IOutMin=[]  IOutMax=[]  DOutMin=[]  DOutMax=[]  NOutMin=[]  NOutMax=[]  KbOutMin=[]  KbOutMax=[]  KtOutMin=[]  KtOutMax=[]  IntegratorOutMin=[]  IntegratorOutMax=[]  FilterOutMin=[]  FilterOutMax=[]  SumOutMin=[]  SumOutMax=[]  SumI1OutMin=[]  SumI1OutMax=[]  SumI2OutMin=[]  SumI2OutMax=[]  SumI3OutMin=[]  SumI3OutMax=[]  SumDOutMin=[]  SumDOutMax=[]  SaturationOutMin=[]  SaturationOutMax=[]  IntegratorContinuousStateAttributes=''  IntegratorStateMustResolveToSignalObject=off  IntegratorRTWStateStorageClass=Auto  FilterContinuousStateAttributes=''  FilterStateMustResolveToSignalObject=off  FilterRTWStateStorageClass=Auto  DifferentiatorICPrevScaledInput=0  DifferentiatorOutMin=[]  DifferentiatorOutMax=[]  UseFilter=on
  PI_Ireg1 : Scope
      settings: YMin=-0.25  YMax=0.45
  Rff : Gain  Gain=RLff(1)  SaturateOnIntegerOverflow=on  OutDataTypeStr=Inherit: Same as input  ParamDataTypeStr=Inherit: Same as input
  "Rff " : Gain  Gain=RLff(1)  SaturateOnIntegerOverflow=on  OutDataTypeStr=Inherit: Same as input  ParamDataTypeStr=Inherit: Same as input
  Saturation : Saturate  UpperLimit=1.5  LowerLimit=-1.5
  Sum : Sum  Inputs=|-+
  VdVq_conv : Outport
  wires:
  Add3/1 -> Mux/2
  Demux/2 -> Add3/1
  Add1/1 -> Mux/1  "Feedforward"
  Lff/1 -> Add3/3
  Rff/1 -> Add3/2
  Demux1/2 -> Rff/1, "Lff  "/1
  "Lff  "/1 -> Add1/3
  Demux1/1 -> Lff/1, "Rff "/1
  "Rff "/1 -> Add1/2
  Demux/1 -> Add1/1
  VdVq/1 -> Demux/1
  Saturation/1 -> VdVq_conv/1
  Add2/1 -> Saturation/1
  IdIq/1 -> Sum/1
  IdIq_ref/1 -> Demux1/1, Sum/2
  Sum/1 -> PI/1
  PI/1 -> Add2/1, PI_Ireg1/1  "PI"
  Mux/1 -> Add2/2

== system boost_and_two_level__1_sm_ehs/SM_eHS/source_and_gates/Inverter Control/MPPT  Parameters ==
  note: Upper limit for Vdc_ref (Dmax)
  note: Increment value used to increase/decrease Vdc_ref (DeltaD)
  note: Initial value for Vdc_ref output (Dinit)
  note: Lower limit for Vdc_ref (Dmax)
  note: Parameters for Perturb and Observe Algorithm:
  Iph_ : Constant  Value=Vdc_ref_Init
  Iph_1 : Constant  Value=Limits_MPPT(1)
  Iph_2 : Constant  Value=Limits_MPPT(2)
  Iph_3 : Constant  Value=Increment_MPPT
  Mux : Mux
  Param : Outport
  wires:
  Iph_/1 -> Mux/1
  Iph_1/1 -> Mux/2
  Iph_2/1 -> Mux/3
  Iph_3/1 -> Mux/4
  Mux/1 -> Param/1

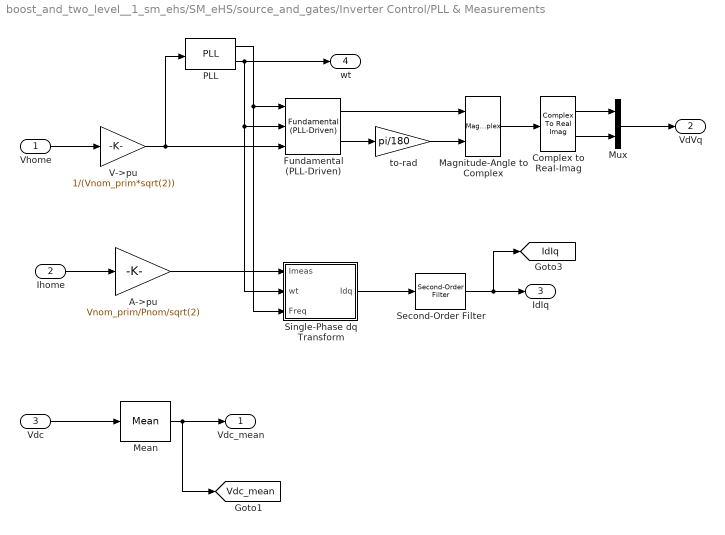
== system boost_and_two_level__1_sm_ehs/SM_eHS/source_and_gates/Inverter Control/PLL & Measurements ==
  Vhome : Inport
  Ihome : Inport  Port=2
  Vdc : Inport  Port=3
  A->pu : Gain  Gain=Vnom_prim/Pnom/sqrt(2)  SaturateOnIntegerOverflow=on  OutDataTypeStr=Inherit: Same as input  ParamDataTypeStr=Inherit: Same as input
  Complex to Real-Imag : ComplexToRealImag
  Fundamental (PLL-Driven) : powerlib_meascontrol/Measurements/Fundamental (PLL-Driven)  Finit=Fnom  Fmin=45  InInit=[1, 0]  Ts=Ts_Control
  Magnitude-Angle to Complex : MagnitudeAngleToComplex
  Mean : powerlib_meascontrol/Measurements/Mean  Freq=Fnom  Vinit=Vdc_ref_Init  Ts=Ts_Control
  Mux : Mux  Inputs=2
  PLL : powerlib_meascontrol/PLL/PLL  Fmin=40  Par_Init=[0, Fnom]  ParK=[180, 3200, 1]  TcD=1e-4  MaxRateChangeFreq=12  FilterCutOffFreq=25  Ts=Ts_Control  AGC=on
  Second-Order Filter : powerlib_meascontrol/Filters/Second-Order Filter  FilterType=Lowpass  Fo=2000  Zeta=1  Ts=Ts_Control  Initialize=on  Vac_Init="[0,  0,  60;0,0,60]"  Vdc_Init=[0.9 0]  PlotResponse=off  FreqRange=[0, 500, 1]
  Single-Phase dq Transform : Subsystem
  V->pu : Gain  Gain=1/(Vnom_prim*sqrt(2))  SaturateOnIntegerOverflow=on  OutDataTypeStr=Inherit: Same as input  ParamDataTypeStr=Inherit: Same as input
  to-rad : Gain  Gain=pi/180
  Vdc_mean : Outport
  VdVq : Outport  Port=2
  IdIq : Outport  Port=3
  wt : Outport  Port=4
  tag scope: IdIq=global, Vdc_mean=global
  wires:
  Mean/1 -> Vdc_mean/1, [Vdc_mean]
  Vdc/1 -> Mean/1
  to-rad/1 -> Magnitude-Angle to Complex/2
  Mux/1 -> VdVq/1
  Complex to Real-Imag/2 -> Mux/2
  Complex to Real-Imag/1 -> Mux/1
  Magnitude-Angle to Complex/1 -> Complex to Real-Imag/1
  Fundamental (PLL-Driven)/2 -> to-rad/1
  Fundamental (PLL-Driven)/1 -> Magnitude-Angle to Complex/1
  A->pu/1 -> Single-Phase dq Transform/1(Imeas)
  PLL/1 -> Single-Phase dq Transform/3(Freq), Fundamental (PLL-Driven)/1
  PLL/2 -> wt/1, Fundamental (PLL-Driven)/2, Single-Phase dq Transform/2(wt)
  Ihome/1 -> A->pu/1
  Vhome/1 -> V->pu/1
  V->pu/1 -> Fundamental (PLL-Driven)/3, PLL/1
  Single-Phase dq Transform/1(Idq) -> Second-Order Filter/1
  Second-Order Filter/1 -> [IdIq], IdIq/1

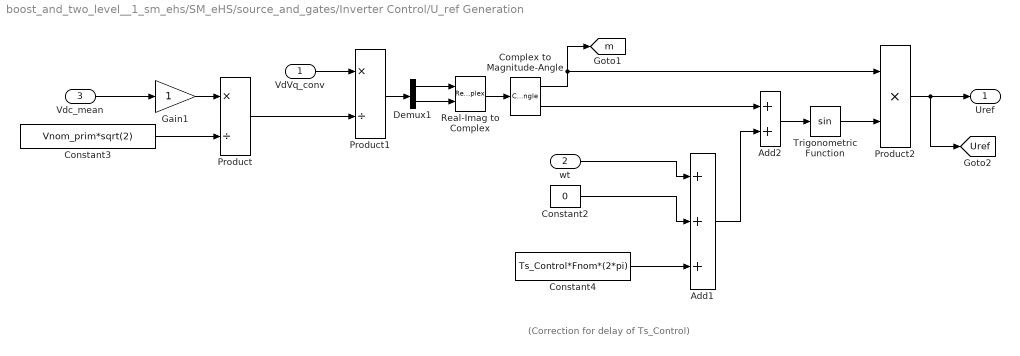
== system boost_and_two_level__1_sm_ehs/SM_eHS/source_and_gates/Inverter Control/U_ref Generation  ==
  note: (Correction for delay of Ts_Control)
  VdVq_conv : Inport
  wt : Inport  Port=2
  Vdc_mean : Inport  Port=3
  Add1 : Sum  Inputs=+++
  Add2 : Sum
  Complex to Magnitude-Angle : ComplexToMagnitudeAngle
  Constant2 : Constant  Value=0
  Constant3 : Constant  Value=Vnom_prim*sqrt(2)
  Constant4 : Constant  Value=Ts_Control*Fnom*(2*pi)
  Demux1 : Demux  Outputs=2
  Gain1 : Gain
  Product : Product  Inputs=*/  RndMeth=Zero
  Product1 : Product  Inputs=*/  RndMeth=Zero
  Product2 : Product  Inputs=**  RndMeth=Zero
  Real-Imag to Complex : RealImagToComplex
  Trigonometric Function : Trigonometry
  Uref : Outport
  tag scope: Uref=global, m=global
  wires:
  VdVq_conv/1 -> Product1/1
  Product2/1 -> Uref/1, [Uref]
  Vdc_mean/1 -> Gain1/1
  Constant4/1 -> Add1/3
  wt/1 -> Add1/1
  Trigonometric Function/1 -> Product2/2
  Complex to Magnitude-Angle/1 -> [m], Product2/1
  Add2/1 -> Trigonometric Function/1
  Add1/1 -> Add2/2
  Complex to Magnitude-Angle/2 -> Add2/1
  Product/1 -> Product1/2
  Constant3/1 -> Product/2
  Constant2/1 -> Add1/2
  Demux1/2 -> Real-Imag to Complex/2
  Demux1/1 -> Real-Imag to Complex/1
  Real-Imag to Complex/1 -> Complex to Magnitude-Angle/1
  Gain1/1 -> Product/1
  Product1/1 -> Demux1/1

== system boost_and_two_level__1_sm_ehs/SM_eHS/source_and_gates/Inverter Control/VDC Regulator ==
  Vdc_ref : Inport  PortDimensions=1
  Vdc_mean : Inport  Port=2  PortDimensions=1
  PI : simulink/Continuous/PID Controller  Controller=PI  TimeDomain=Discrete-time  SampleTime=Ts_Control  IntegratorMethod=Trapezoidal  FilterMethod=Forward Euler  Form=Parallel  P=Kp_VDCreg  I=Ki_VDCreg  D=0  N=100  InitialConditionSource=internal  InitialConditionForIntegrator=0.9226  InitialConditionForFilter=0  ExternalReset=none  LimitOutput=on  UpperSaturationLimit=1.5  LowerSaturationLimit=-1.5  LinearizeAsGain=off  AntiWindupMode=none  Kb=1  TrackingMode=off  Kt=1  PParamMin=[]  PParamMax=[]  IParamMin=[]  IParamMax=[]  DParamMin=[]  DParamMax=[]  NParamMin=[]  NParamMax=[]  KbParamMin=[]  KbParamMax=[]  KtParamMin=[]  KtParamMax=[]  POutMin=[]  POutMax=[]  IOutMin=[]  IOutMax=[]  DOutMin=[]  DOutMax=[]  NOutMin=[]  NOutMax=[]  KbOutMin=[]  KbOutMax=[]  KtOutMin=[]  KtOutMax=[]  IntegratorOutMin=[]  IntegratorOutMax=[]  FilterOutMin=[]  FilterOutMax=[]  SumOutMin=[]  SumOutMax=[]  SumI1OutMin=[]  SumI1OutMax=[]  SumI2OutMin=[]  SumI2OutMax=[]  SumI3OutMin=[]  SumI3OutMax=[]  SumDOutMin=[]  SumDOutMax=[]  SaturationOutMin=[]  SaturationOutMax=[]  IntegratorContinuousStateAttributes=''  IntegratorStateMustResolveToSignalObject=off  IntegratorRTWStateStorageClass=Auto  FilterContinuousStateAttributes=''  FilterStateMustResolveToSignalObject=off  FilterRTWStateStorageClass=Auto  DifferentiatorICPrevScaledInput=0  DifferentiatorOutMin=[]  DifferentiatorOutMax=[]  UseFilter=on
  Rtot_pu2 : Gain  Gain=1/Vnom_dc  SaturateOnIntegerOverflow=on  OutDataTypeStr=Inherit: Same as input  ParamDataTypeStr=Inherit: Same as input
  Sum : Sum  Inputs=|+-
  Id_ref : Outport  InitialOutput=0
  tag scope: Id_ref=global, Vdc_ref=global
  wires:
  Rtot_pu2/1 -> PI/1
  Vdc_ref/1 -> Sum/2, [Vdc_ref]
  Vdc_mean/1 -> Sum/1
  Sum/1 -> Rtot_pu2/1
  PI/1 -> Id_ref/1, [Id_ref]

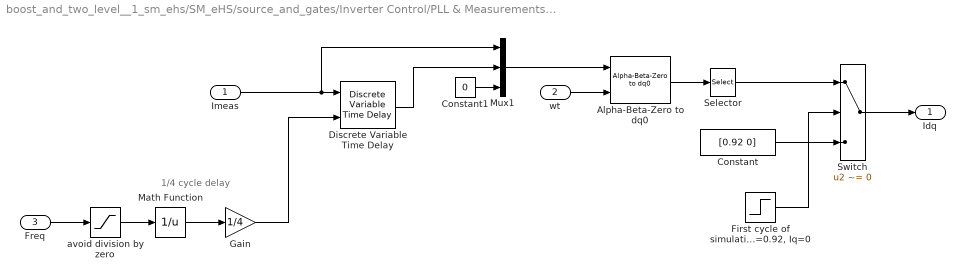
== system boost_and_two_level__1_sm_ehs/SM_eHS/source_and_gates/Inverter Control/PLL & Measurements/Single-Phase dq Transform ==
  note: 1/4 cycle delay
  Imeas : Inport
  wt : Inport  Port=2
  Freq : Inport  Port=3
  Alpha-Beta-Zero to dq0 : powerlib_meascontrol/Transformations/Alpha-Beta-Zero to dq0  Alignment=90 degrees behind phase A axis
  Constant : Constant  Value=[0.92 0]
  Constant1 : Constant  Value=0
  Discrete Variable Time Delay : powerlib_meascontrol/Additional Components/Discrete Variable Time Delay  MaxDelay=1  InitialValue=0  Ts=Ts_Control  DFT=on
  "First cycle of simulation Id=0.92, Iq=0" : Step  Time=1/Fnom  SampleTime=Ts_Control
  Gain : Gain  Gain=1/4
  Math Function : Math  Operator=reciprocal  SaturateOnIntegerOverflow=on
  Mux1 : Mux  Inputs=3
  Selector : Selector  InputPortWidth=3  Indices=[1 2]
  Switch : Switch  Criteria=u2 ~= 0
  avoid division by zero : Saturate  UpperLimit=70  LowerLimit=40
  Idq : Outport
  wires:
  Constant1/1 -> Mux1/3
  Discrete Variable Time Delay/1 -> Mux1/2
  Mux1/1 -> Alpha-Beta-Zero to dq0/1
  Imeas/1 -> Discrete Variable Time Delay/1, Mux1/1
  wt/1 -> Alpha-Beta-Zero to dq0/2
  Alpha-Beta-Zero to dq0/1 -> Selector/1
  Freq/1 -> avoid division by zero/1
  avoid division by zero/1 -> Math Function/1
  Math Function/1 -> Gain/1
  Gain/1 -> Discrete Variable Time Delay/2
  Selector/1 -> Switch/1
  Switch/1 -> Idq/1
  Constant/1 -> Switch/3
  "First cycle of simulation Id=0.92, Iq=0"/1 -> Switch/2

== matlab function SM_eHS/source_and_gates/MATLAB Function ==
  data: Vb input double; Iph output double; G input double; Ta input double; Ncell input double; Isc input double; Voc input double; Ksc input double; Io output double
function [Iph, Io] = PVpanel_new(Vb, G, Ta, Ncell, Isc, Voc, Ksc)

    toKelvin = 273;
    Ksc = Ksc / 100;
    G_ref = 1000;
    Ta_ref = 25 + toKelvin;
    Ta = Ta + toKelvin;
    deltaT = Ta - Ta_ref;
    k = 1.381e-23;
    q = 1.6e-19;
    eg = 1.12;                  % bandgap energy(1.12 eV)
    A = 1.3;                    % ideal factor
    a = Ncell * k * A * Ta / q;
    a_ref = Ncell * k * A * Ta_ref / q;
    Iph_ref = Isc;
    Voc_ref = Voc;
    Iph = G / G_ref * Iph_ref * (1 + Ksc * deltaT);
    Io_ref = Iph_ref / (exp(Voc_ref / a_ref) - 1);
    Io = Io_ref * (Ta / Ta_ref)^3 * ...
        exp((q * eg / A / k) * (1/Ta_ref - 1/Ta));
    Io = Io * (exp(Vb / a) - 1);

end

== matlab function SM_eHS/source_and_gates/Inverter Control/MPPT Controller using Perturbe & Observe technique  ==
  settings: updateMethod=DISCRETE  sampleTime=Ts_Control
  data: Param input double; Enabled input double; V input double; I input double; D output double
function D  = PandO(Param, Enabled, V, I)

% MPPT controller based on the Perturb & Observe algorithm.

% D output = Reference for DC link voltage (Vdc_ref) 
%
% Enabled input = 1 to enable the MPPT controller
% V input = PV array terminal voltage (V)
% I input = PV array current (A)
%
% Param input:
Dinit = Param(1);  %Initial value for Vdc_ref
Dmax = Param(2);   %Maximum value for Vdc_ref
Dmin = Param(3);   %Minimum value for Vdc_ref
deltaD = Param(4); %Increment value used to increase/decrease Vdc_ref
%  

persistent Vold Pold Dold;

dataType = 'double';

if isempty(Vold)
    Vold=0;
    Pold=0;
    Dold=Dinit;
end
P= V*I;
dV= V - Vold;
dP= P - Pold;

if dP ~= 0 & Enabled ~=0
    if dP < 0
        if dV < 0
            D = Dold + deltaD;
        else
            D = Dold - deltaD;
        end
    else
        if dV < 0
            D = Dold - deltaD;
        else
            D = Dold + deltaD;
        end    
    end
else D=Dold;
end

if D >= Dmax | D<= Dmin
    D=Dold;
end

Dold=D;
Vold=V;
Pold=P;
